simulink model "que3w3"  (R2020b)
settings: Solver=VariableStepAuto  StartTime=0.0  StopTime=10.0  RelTol=1e-3
undefined symbols (not defined in the file): ctrl, g, I, Kf, m, mu, PBmax, Rr, sigbuilder_block, slip, TB, v0
settings Model: DataDictionary=data_dict.sldd  Creator=ANUJA  LastModifiedBy=ANUJA

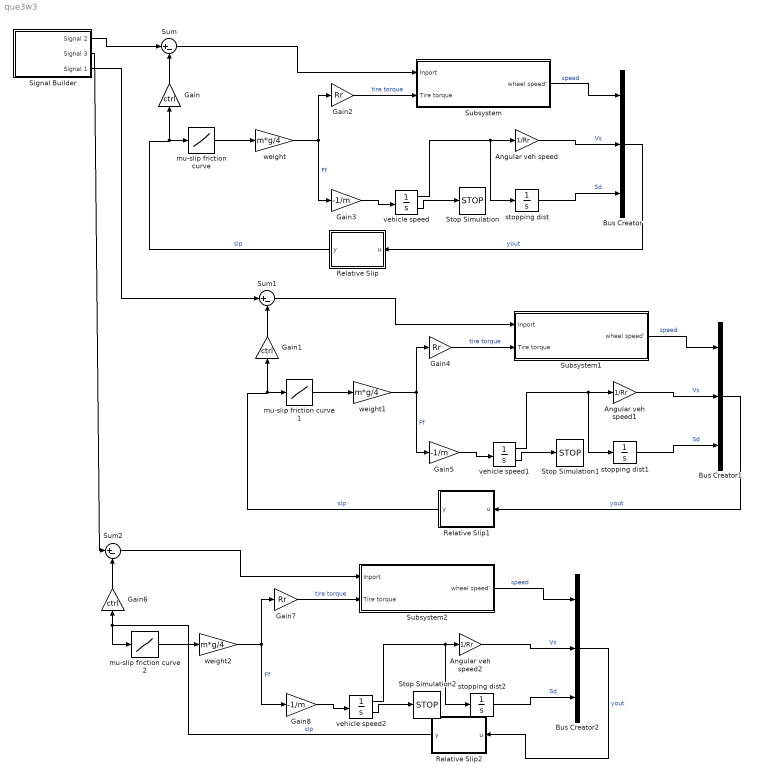
== system que3w3 ==
  Angular veh speed : Gain  Gain=1/Rr
  Angular veh speed1 : Gain  Gain=1/Rr
  Angular veh speed2 : Gain  Gain=1/Rr
  Bus Creator : BusCreator  Inputs=3
  Bus Creator1 : BusCreator  Inputs=3
  Bus Creator2 : BusCreator  Inputs=3
  Gain : Gain  Gain=ctrl
  Gain1 : Gain  Gain=ctrl
  Gain2 : Gain  Gain=Rr
  Gain3 : Gain  Gain=-1/m
  Gain4 : Gain  Gain=Rr
  Gain5 : Gain  Gain=-1/m
  Gain6 : Gain  Gain=ctrl
  Gain7 : Gain  Gain=Rr
  Gain8 : Gain  Gain=-1/m
  Relative Slip : MATLAB Function  TreatAsAtomicUnit=on
  Relative Slip1 : MATLAB Function  TreatAsAtomicUnit=on
  Relative Slip2 : MATLAB Function  TreatAsAtomicUnit=on
  Signal Builder : Subsystem  Tag=STV Subsys  LoadFcn=sigbuilder_block('load',[437.6 153 550.4 359.25 ]);  StartFcn=sigbuilder_block('start');  StopFcn=sigbuilder_block('stop');  ClipboardFcn=sigbuilder_block('clipboard');  mask(Sigbuilder block){tuvar=[0:10]}
      mask help: Simulink:masks:SigbuilderBlock_MD
      mask init:
      | if ~strcmp(get_param(bdroot(gcbh),'SimulationStatus'),'stopped') tuvar = sigbuilder_block('maskInit'); end
      settings: CopyFcn=sigbuilder_block('copy');  DeleteFcn=sigbuilder_block('delete');  ModelCloseFcn=sigbuilder_block('modelClose');  PreSaveFcn=sigbuilder_block('preSave');  PauseFcn=sigbuilder_block('pause');  ContinueFcn=sigbuilder_block('continue');  NameChangeFcn=sigbuilder_block('namechange');  OpenFcn=sigbuilder_block('open',[437.6 153 550.4 359.25 ]);  CloseFcn=sigbuilder_block('close');
      mask Display: plot(0, 0, 100, 100,[2, 2, 32, 32, 2], [68, 8, 8, 68, 68],[32, 2], [38, 38], [32, 19, 2],[53, 60, 44], [32, 17, 17, 2],[16, 16, 31, 31]);txt = getActiveGroup(gcbh);text(2, 100, txt,'verticalAlignment', 'top');
  Stop Simulation : Stop
  Stop Simulation1 : Stop
  Stop Simulation2 : Stop
  Subsystem : Subsystem
  Subsystem1 : Subsystem
  Subsystem2 : Subsystem
  Sum : Sum  Inputs=|+-
  Sum1 : Sum  Inputs=|+-
  Sum2 : Sum  Inputs=|+-
  "mu-slip friction curve " : Lookup_n-D  NumberOfTableDimensions=1  BreakpointsForDimension1=slip  Table=mu  InternalRulePriority=Speed  RndMeth=Simplest  InputSameDT=on
  mu-slip friction curve 1 : Lookup_n-D  NumberOfTableDimensions=1  BreakpointsForDimension1=slip  Table=mu  InternalRulePriority=Speed  RndMeth=Simplest  InputSameDT=on
  mu-slip friction curve 2 : Lookup_n-D  NumberOfTableDimensions=1  BreakpointsForDimension1=slip  Table=mu  InternalRulePriority=Speed  RndMeth=Simplest  InputSameDT=on
  stopping dist : Integrator
  stopping dist1 : Integrator
  stopping dist2 : Integrator
  vehicle speed : Integrator  InitialCondition=v0  LimitOutput=on  UpperSaturationLimit=1000  LowerSaturationLimit=0  ShowSaturationPort=on
  vehicle speed1 : Integrator  InitialCondition=v0  LimitOutput=on  UpperSaturationLimit=1000  LowerSaturationLimit=0  ShowSaturationPort=on
  vehicle speed2 : Integrator  InitialCondition=v0  LimitOutput=on  UpperSaturationLimit=1000  LowerSaturationLimit=0  ShowSaturationPort=on
  weight : Gain  Gain=m*g/4
  weight1 : Gain  Gain=m*g/4
  weight2 : Gain  Gain=m*g/4
  wires:
  Gain6/1 -> Sum2/2
  Relative Slip2/1(y) -> mu-slip friction curve 2/1, Gain6/1  "slp"
  Bus Creator2/1 -> Relative Slip2/1(u)  "yout"
  Gain7/1 -> Subsystem2/2(Tire torque)  "tire torque"
  vehicle speed1/2 -> Stop Simulation1/1
  Subsystem/1(wheel speed') -> Bus Creator/1  "speed"
  vehicle speed/1 -> stopping dist/1, Angular veh speed/1
  vehicle speed2/2 -> Stop Simulation2/1
  Bus Creator1/1 -> Relative Slip1/1(u)  "yout"
  weight2/1 -> Gain8/1, Gain7/1  "Ff"
  Gain8/1 -> vehicle speed2/1
  stopping dist/1 -> Bus Creator/3  "Sd"
  Angular veh speed/1 -> Bus Creator/2  "Vs"
  stopping dist2/1 -> Bus Creator2/3  "Sd"
  Angular veh speed2/1 -> Bus Creator2/2  "Vs"
  Sum2/1 -> Subsystem2/1(Inport)
  Subsystem2/1(wheel speed') -> Bus Creator2/1  "speed"
  Gain3/1 -> vehicle speed/1
  Gain/1 -> Sum/2
  vehicle speed/2 -> Stop Simulation/1
  Gain2/1 -> Subsystem/2(Tire torque)  "tire torque"
  Gain4/1 -> Subsystem1/2(Tire torque)  "tire torque"
  mu-slip friction curve 2/1 -> weight2/1
  Bus Creator/1 -> Relative Slip/1(u)  "yout"
  Relative Slip/1(y) -> "mu-slip friction curve "/1, Gain/1  "slp"
  Signal Builder/2(Signal 3) -> Sum2/1
  stopping dist1/1 -> Bus Creator1/3  "Sd"
  weight1/1 -> Gain5/1, Gain4/1  "Ff"
  Gain1/1 -> Sum1/2
  mu-slip friction curve 1/1 -> weight1/1
  Sum1/1 -> Subsystem1/1(Inport)
  "mu-slip friction curve "/1 -> weight/1
  Gain5/1 -> vehicle speed1/1
  Relative Slip1/1(y) -> mu-slip friction curve 1/1, Gain1/1  "slp"
  vehicle speed2/1 -> stopping dist2/1, Angular veh speed2/1
  vehicle speed1/1 -> stopping dist1/1, Angular veh speed1/1
  Angular veh speed1/1 -> Bus Creator1/2  "Vs"
  weight/1 -> Gain3/1, Gain2/1  "Ff"
  Sum/1 -> Subsystem/1(Inport)
  Subsystem1/1(wheel speed') -> Bus Creator1/1  "speed"
  Signal Builder/1(Signal 2) -> Sum/1
  Signal Builder/3(Signal 1) -> Sum1/1

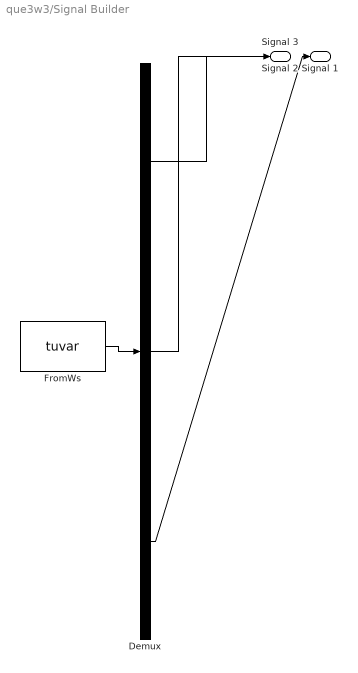
== system que3w3/Signal Builder ==
  Demux : Demux  Tag=STV Demux  Outputs=3
      settings: DisplayOption=none
  FromWs : FromWorkspace  Tag=STV FromWs  VariableName=tuvar
      SigBuilderData=|
      | common.afterFinalStr = 'Extrapolate'
      | common.sampleTime = 0
      | dataSet.timeRange = [0 10]
      | dataSet.name = 'Group 1'
      | sbobj.Groups.Name = 'Group 1'
      | sbobj.Groups.Signals(1).Name = 'Signal 2'
      | sbobj.Groups.Signals(1).XData = [0 3 3 10]
      | sbobj.Groups.Signals(1).YData = [0 0 1.01 0.03]
      | sbobj.Groups.Signals(2).Name = 'Signal 3'
      | sbobj.Groups.Signals(2).XData = [0 4.22 4.22 6.72 6.72 10]
      | sbobj.Groups.Signals(2).YData = [0 0 0.5 0.86 0 0]
      | sbobj.Groups.Signals(3).Name = 'Signal 1'
      | sbobj.Groups.Signals(3).XData = [0 10]
      | sbobj.Groups.Signals(3).YData = [0 0]
  Signal 2 : Outport  Tag=STV Outport
  Signal 3 : Outport  Tag=STV Outport  Port=2
  Signal 1 : Outport  Tag=STV Outport  Port=3
  wires:
  FromWs/1 -> Demux/1
  Demux/1 -> Signal 2/1
  Demux/2 -> Signal 3/1
  Demux/3 -> Signal 1/1

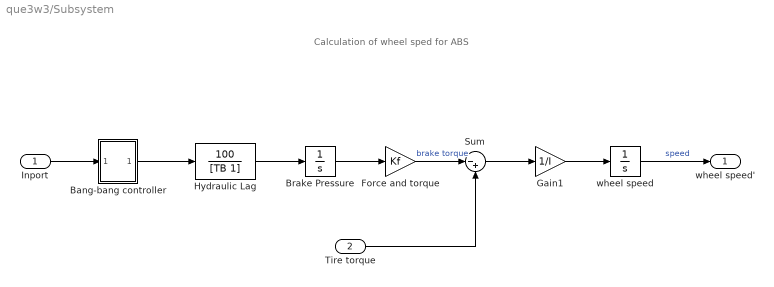
== system que3w3/Subsystem ==
  note: Calculation of wheel sped for ABS
  Inport : Inport
  Tire torque : Inport  Port=2
  Bang-bang controller : Subsystem  mask(Sign){}
      mask help: y = sign(x)
      mask Help: Sign Function:\n\t\t\ty = 1 if x > 0\n\t\t\ty = 0 if x = 0\n\t\t\ty = -1 if x < 0
      mask Display: plot(-50,-50,50,50,[-50,50],[0,0],[0,0],[-50,50],[-40,0],[-30,-30],[0,40],[30,30])
  Brake Pressure : Integrator  LimitOutput=on  UpperSaturationLimit=PBmax  LowerSaturationLimit=0
  Force and torque : Gain  Gain=Kf
  Gain1 : Gain  Gain=1/I
  Hydraulic Lag : TransferFcn  Numerator=[100]  Denominator=[TB 1]
  Sum : Sum  Inputs=|-+
  wheel speed : Integrator  InitialCondition=v0/Rr  LimitOutput=on  UpperSaturationLimit=1000  LowerSaturationLimit=0
  wheel speed' : Outport
  wires:
  Brake Pressure/1 -> Force and torque/1
  Sum/1 -> Gain1/1
  Bang-bang controller/1(out_1) -> Hydraulic Lag/1
  wheel speed/1 -> wheel speed'/1  "speed"
  Tire torque/1 -> Sum/2
  Gain1/1 -> wheel speed/1
  Inport/1 -> Bang-bang controller/1(in_1)
  Hydraulic Lag/1 -> Brake Pressure/1
  Force and torque/1 -> Sum/1  "brake torque"

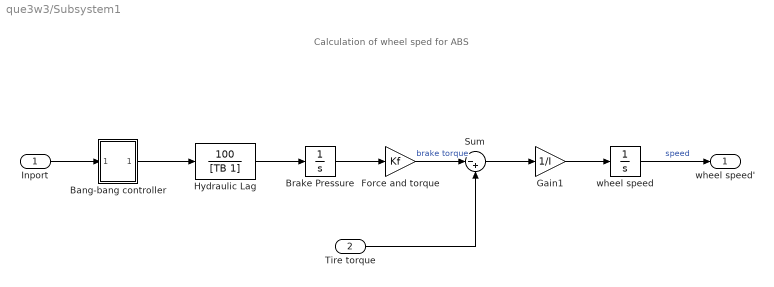
== system que3w3/Subsystem1 ==
  note: Calculation of wheel sped for ABS
  Inport : Inport
  Tire torque : Inport  Port=2
  Bang-bang controller : Subsystem  mask(Sign){}
      mask help: y = sign(x)
      mask Help: Sign Function:\n\t\t\ty = 1 if x > 0\n\t\t\ty = 0 if x = 0\n\t\t\ty = -1 if x < 0
      mask Display: plot(-50,-50,50,50,[-50,50],[0,0],[0,0],[-50,50],[-40,0],[-30,-30],[0,40],[30,30])
  Brake Pressure : Integrator  LimitOutput=on  UpperSaturationLimit=PBmax  LowerSaturationLimit=0
  Force and torque : Gain  Gain=Kf
  Gain1 : Gain  Gain=1/I
  Hydraulic Lag : TransferFcn  Numerator=[100]  Denominator=[TB 1]
  Sum : Sum  Inputs=|-+
  wheel speed : Integrator  InitialCondition=v0/Rr  LimitOutput=on  UpperSaturationLimit=1000  LowerSaturationLimit=0
  wheel speed' : Outport
  wires:
  Brake Pressure/1 -> Force and torque/1
  Sum/1 -> Gain1/1
  Bang-bang controller/1(out_1) -> Hydraulic Lag/1
  wheel speed/1 -> wheel speed'/1  "speed"
  Tire torque/1 -> Sum/2
  Gain1/1 -> wheel speed/1
  Inport/1 -> Bang-bang controller/1(in_1)
  Hydraulic Lag/1 -> Brake Pressure/1
  Force and torque/1 -> Sum/1  "brake torque"

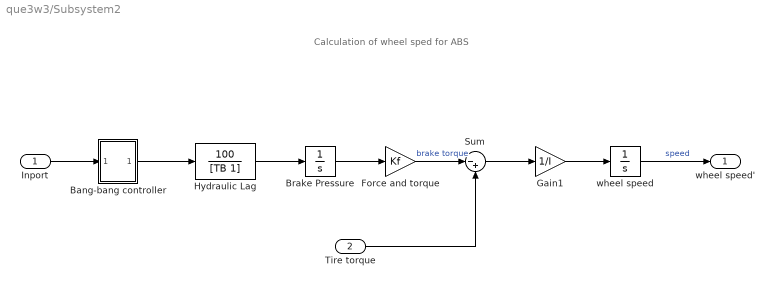
== system que3w3/Subsystem2 ==
  note: Calculation of wheel sped for ABS
  Inport : Inport
  Tire torque : Inport  Port=2
  Bang-bang controller : Subsystem  mask(Sign){}
      mask help: y = sign(x)
      mask Help: Sign Function:\n\t\t\ty = 1 if x > 0\n\t\t\ty = 0 if x = 0\n\t\t\ty = -1 if x < 0
      mask Display: plot(-50,-50,50,50,[-50,50],[0,0],[0,0],[-50,50],[-40,0],[-30,-30],[0,40],[30,30])
  Brake Pressure : Integrator  LimitOutput=on  UpperSaturationLimit=PBmax  LowerSaturationLimit=0
  Force and torque : Gain  Gain=Kf
  Gain1 : Gain  Gain=1/I
  Hydraulic Lag : TransferFcn  Numerator=[100]  Denominator=[TB 1]
  Sum : Sum  Inputs=|-+
  wheel speed : Integrator  InitialCondition=v0/Rr  LimitOutput=on  UpperSaturationLimit=1000  LowerSaturationLimit=0
  wheel speed' : Outport
  wires:
  Brake Pressure/1 -> Force and torque/1
  Sum/1 -> Gain1/1
  Bang-bang controller/1(out_1) -> Hydraulic Lag/1
  wheel speed/1 -> wheel speed'/1  "speed"
  Tire torque/1 -> Sum/2
  Gain1/1 -> wheel speed/1
  Inport/1 -> Bang-bang controller/1(in_1)
  Hydraulic Lag/1 -> Brake Pressure/1
  Force and torque/1 -> Sum/1  "brake torque"

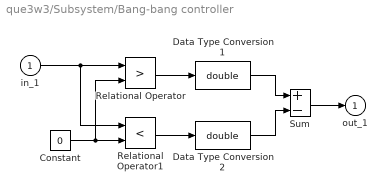
== system que3w3/Subsystem/Bang-bang controller ==
  in_1 : Inport
  Constant : Constant  Value=0
  Data Type Conversion1 : DataTypeConversion  OutDataTypeStr=double  SaturateOnIntegerOverflow=on  RndMeth=Zero
  Data Type Conversion2 : DataTypeConversion  OutDataTypeStr=double  SaturateOnIntegerOverflow=on  RndMeth=Zero
  Relational Operator : RelationalOperator  Operator=>  OutDataTypeStr=boolean  RndMeth=Nearest  InputSameDT=on
  Relational Operator1 : RelationalOperator  Operator=<  OutDataTypeStr=boolean  RndMeth=Nearest  InputSameDT=on
  Sum : Sum  Inputs=+-  InputSameDT=on  SaturateOnIntegerOverflow=on  OutDataTypeStr=Inherit: Same as first input
  out_1 : Outport  InitialOutput=0  VectorParamsAs1DForOutWhenUnconnected=off
  wires:
  Data Type Conversion2/1 -> Sum/2
  Data Type Conversion1/1 -> Sum/1
  Sum/1 -> out_1/1
  Relational Operator/1 -> Data Type Conversion1/1
  Relational Operator1/1 -> Data Type Conversion2/1
  Constant/1 -> Relational Operator/2, Relational Operator1/2
  in_1/1 -> Relational Operator1/1, Relational Operator/1

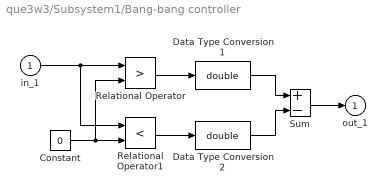
== system que3w3/Subsystem1/Bang-bang controller ==
  in_1 : Inport
  Constant : Constant  Value=0
  Data Type Conversion1 : DataTypeConversion  OutDataTypeStr=double  SaturateOnIntegerOverflow=on  RndMeth=Zero
  Data Type Conversion2 : DataTypeConversion  OutDataTypeStr=double  SaturateOnIntegerOverflow=on  RndMeth=Zero
  Relational Operator : RelationalOperator  Operator=>  OutDataTypeStr=boolean  RndMeth=Nearest  InputSameDT=on
  Relational Operator1 : RelationalOperator  Operator=<  OutDataTypeStr=boolean  RndMeth=Nearest  InputSameDT=on
  Sum : Sum  Inputs=+-  InputSameDT=on  SaturateOnIntegerOverflow=on  OutDataTypeStr=Inherit: Same as first input
  out_1 : Outport  InitialOutput=0  VectorParamsAs1DForOutWhenUnconnected=off
  wires:
  Data Type Conversion2/1 -> Sum/2
  Data Type Conversion1/1 -> Sum/1
  Sum/1 -> out_1/1
  Relational Operator/1 -> Data Type Conversion1/1
  Relational Operator1/1 -> Data Type Conversion2/1
  Constant/1 -> Relational Operator/2, Relational Operator1/2
  in_1/1 -> Relational Operator1/1, Relational Operator/1

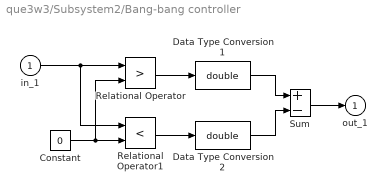
== system que3w3/Subsystem2/Bang-bang controller ==
  in_1 : Inport
  Constant : Constant  Value=0
  Data Type Conversion1 : DataTypeConversion  OutDataTypeStr=double  SaturateOnIntegerOverflow=on  RndMeth=Zero
  Data Type Conversion2 : DataTypeConversion  OutDataTypeStr=double  SaturateOnIntegerOverflow=on  RndMeth=Zero
  Relational Operator : RelationalOperator  Operator=>  OutDataTypeStr=boolean  RndMeth=Nearest  InputSameDT=on
  Relational Operator1 : RelationalOperator  Operator=<  OutDataTypeStr=boolean  RndMeth=Nearest  InputSameDT=on
  Sum : Sum  Inputs=+-  InputSameDT=on  SaturateOnIntegerOverflow=on  OutDataTypeStr=Inherit: Same as first input
  out_1 : Outport  InitialOutput=0  VectorParamsAs1DForOutWhenUnconnected=off
  wires:
  Data Type Conversion2/1 -> Sum/2
  Data Type Conversion1/1 -> Sum/1
  Sum/1 -> out_1/1
  Relational Operator/1 -> Data Type Conversion1/1
  Relational Operator1/1 -> Data Type Conversion2/1
  Constant/1 -> Relational Operator/2, Relational Operator1/2
  in_1/1 -> Relational Operator1/1, Relational Operator/1

== matlab function que3w3/Relative Slip ==
  data: u input; y output
function y = fcn(u)

y = 1.0 - u(1)/(u(2) + (u(2)==0)*eps);

== matlab function que3w3/Relative Slip2 ==
  data: u input; y output
function y = fcn(u)

y = 1.0 - u(1)/(u(2) + (u(2)==0)*eps);

== matlab function que3w3/Relative Slip1 ==
  data: u input; y output
function y = fcn(u)

y = 1.0 - u(1)/(u(2) + (u(2)==0)*eps);
